simulink model "simulacion_4_1"  (R2021b)
settings: Solver=VariableStepAuto  StartTime=0.0  StopTime=10.0  RelTol=1e-3
libraries: spsSeriesRLCBranchLib x6, spsACVoltageSourceLib x3, spsGroundLib x1, spsPower3phPhasorLib x1, spsPowerPhasorLib x1, spsThreePhaseVIMeasurementLib x1, spspowerguiLib x1
settings Model: Creator=Roberto  LastModifiedBy=Roberto

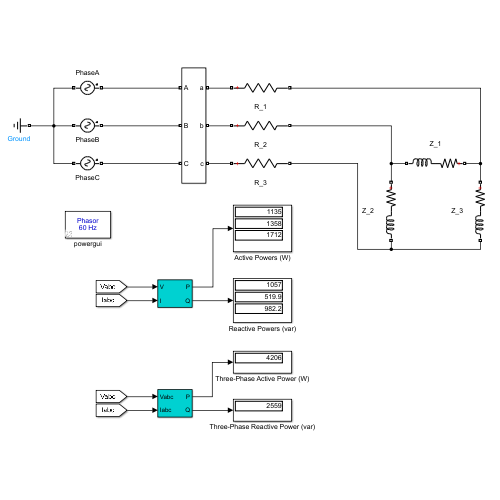
[thumbnail: Simulink's stored preview of the top-level diagram]
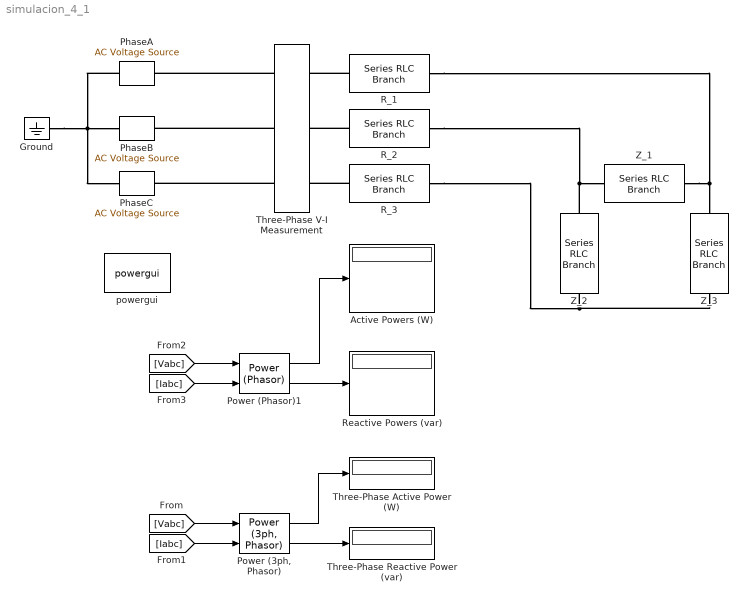
== system simulacion_4_1 ==
  Active Powers (W) : Display
  Ground : spsGroundLib/Ground  LConnTagsString=a
  PhaseA : spsACVoltageSourceLib/AC Voltage Source  Amplitude=100  Phase=0  Frequency=60  SampleTime=0  Measurements=None  BusType=swing  Pref=10e3  Qref=0  Qmin=-inf  Qmax=+inf
  PhaseB : spsACVoltageSourceLib/AC Voltage Source  Amplitude=100  Phase=-120  Frequency=60  SampleTime=0  Measurements=None  BusType=swing  Pref=10e3  Qref=0  Qmin=-inf  Qmax=+inf
  PhaseC : spsACVoltageSourceLib/AC Voltage Source  Amplitude=100  Phase=+120  Frequency=60  SampleTime=0  Measurements=None  BusType=swing  Pref=10e3  Qref=0  Qmin=-inf  Qmax=+inf
  "Power (3ph, Phasor)" : spsPower3phPhasorLib/Power (3ph, Phasor)
      settings: SourceProductBaseCode=PS
  Power (Phasor)1 : spsPowerPhasorLib/Power (Phasor)
      settings: SourceProductBaseCode=PS
  R_1 : spsSeriesRLCBranchLib/Series RLC Branch  LConnTagsString=__new0  RConnTagsString=__new0  BranchType=R  Resistance=0.5  Inductance=1e-3  SetiL0=off  InitialCurrent=0  Capacitance=1e-6  Setx0=off  InitialVoltage=0  Measurements=None
  R_2 : spsSeriesRLCBranchLib/Series RLC Branch  LConnTagsString=__new0  RConnTagsString=__new0  BranchType=R  Resistance=0.5  Inductance=1e-3  SetiL0=off  InitialCurrent=0  Capacitance=1e-6  Setx0=off  InitialVoltage=0  Measurements=None
  R_3 : spsSeriesRLCBranchLib/Series RLC Branch  LConnTagsString=__new0  RConnTagsString=__new0  BranchType=R  Resistance=0.5  Inductance=1e-3  SetiL0=off  InitialCurrent=0  Capacitance=1e-6  Setx0=off  InitialVoltage=0  Measurements=None
  Reactive Powers (var) : Display
  Three-Phase V-I Measurement : spsThreePhaseVIMeasurementLib/Three-Phase V-I Measurement  VoltageMeasurement=phase-to-ground  SetLabelV=on  LabelV=Vabc  Vpu=off  VpuLL=off  CurrentMeasurement=yes  SetLabelI=on  LabelI=Iabc  Ipu=off  Pbase=100e6  Vbase=500e3  OutputType=Complex  PhasorSimulation=on  PSBequivalent=0
  Three-Phase Active Power (W) : Display
  Three-Phase Reactive Power (var) : Display
  Z_1 : spsSeriesRLCBranchLib/Series RLC Branch  LConnTagsString=__new0  RConnTagsString=__new0  BranchType=RL  Resistance=8  Inductance=7/(2*pi*60)  SetiL0=off  InitialCurrent=0  Capacitance=1e-6  Setx0=off  InitialVoltage=0  Measurements=None
  Z_2 : spsSeriesRLCBranchLib/Series RLC Branch  LConnTagsString=__new0  RConnTagsString=__new0  BranchType=RL  Resistance=6  Inductance=3/(2*pi*60)  SetiL0=off  InitialCurrent=0  Capacitance=1e-6  Setx0=off  InitialVoltage=0  Measurements=None
  Z_3 : spsSeriesRLCBranchLib/Series RLC Branch  LConnTagsString=__new0  RConnTagsString=__new0  BranchType=RL  Resistance=5  Inductance=5/(2*pi*60)  SetiL0=off  InitialCurrent=0  Capacitance=1e-6  Setx0=off  InitialVoltage=0  Measurements=None
  powergui : spspowerguiLib/powergui  Priority=1  SimulationMode=Phasor  SampleTime=50e-6  frequency=60  Iterations=50  frequencyindice=60  Pbase=100e6  ErrMax=1e-4  UnitsV=kV  UnitsW=MW  buscounter=0  FunctionMessages=off  echomessages=off  EnableUseOfTLC=off  CurrentSourceSwitches=off  DisableSnubberDevices=off  DisableRonSwitches=off  DisableVfSwitches=off  DisplayEquations=off  AutomaticDiscreteSolvers=off  SolverType=Tustin  Interpol=off  ExternalGateDelay=off  methode=off  Ts=0  x0status=blocks  SPID=off  SwTol=0  HookPort=off  NonlinearTolerance=1e-4  nMaxIteration=100  ContinueOnMaxIteration=off  RestoreLinks=warning  ResistiveCurrentMeasurement=off  Frange=[0:2:500]  Ylog=off  Xlog=on  ShowGrid=off  save=off  variable=ZData  structure=0  ZoomFFT=off  StartTime=0.0  cycles=1  DisplayStyle=1  fundamental=60  FreqAxis=off  MaxFrequency=1000  frequencyindicesteady=1  RmsSteady=1  display=off
  wires:
  Power (Phasor)1/2 -> Reactive Powers (var)/1
  "Power (3ph, Phasor)"/1 -> Three-Phase Active Power (W)/1
  [Iabc] -> Power (Phasor)1/2
  Power (Phasor)1/1 -> Active Powers (W)/1
  [Vabc] -> Power (Phasor)1/1
  [Iabc] -> "Power (3ph, Phasor)"/2
  [Vabc] -> "Power (3ph, Phasor)"/1
  "Power (3ph, Phasor)"/2 -> Three-Phase Reactive Power (var)/1
  connections:
  PhaseA/LConn1 -- PhaseC/LConn1 -- Ground/LConn1 -- PhaseB/LConn1
  R_1/LConn1 -- Three-Phase V-I Measurement/RConn1
  R_2/LConn1 -- Three-Phase V-I Measurement/RConn2
  R_3/LConn1 -- Three-Phase V-I Measurement/RConn3
  Three-Phase V-I Measurement/LConn1 -- PhaseA/RConn1
  Three-Phase V-I Measurement/LConn2 -- PhaseB/RConn1
  Three-Phase V-I Measurement/LConn3 -- PhaseC/RConn1
  Z_2/LConn1 -- Z_1/RConn1 -- R_2/RConn1
  Z_1/LConn1 -- R_1/RConn1 -- Z_3/LConn1
  Z_3/RConn1 -- R_3/RConn1 -- Z_2/RConn1
